simulink model "met_Lap_1_31"  (R2020b)
settings: Solver=VariableStepAuto  StartTime=0.0  StopTime=10.0  RelTol=1e-3
undefined symbols (not defined in the file): b, c, d, x0
libraries: simulink x1
settings Model: Creator=Hyperbook  LastModifiedBy=Hyperbook

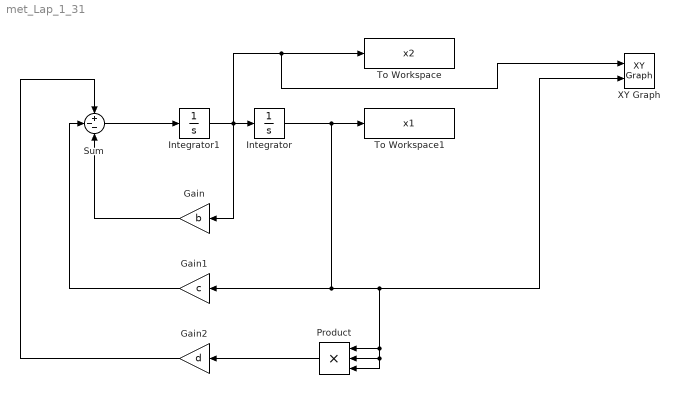
== system met_Lap_1_31 ==
  Gain : Gain  Gain=b
  Gain1 : Gain  Gain=c
  Gain2 : Gain  Gain=d
  Integrator : Integrator  InitialCondition=x0(2)  LimitOutput=on  UpperSaturationLimit=2  LowerSaturationLimit=-2
  Integrator1 : Integrator  InitialCondition=x0(1)  LimitOutput=on  UpperSaturationLimit=2  LowerSaturationLimit=-2
  Product : Product  Inputs=3
  Sum : Sum  Inputs=+--
  To Workspace : ToWorkspace  VariableName=x2  SampleTime=-1
  To Workspace1 : ToWorkspace  VariableName=x1  SampleTime=-1
  XY Graph : simulink/Sinks/XY Graph  xmin=-1  xmax=1  ymin=-1  ymax=1  st=-1
  wires:
  Integrator/1 -> XY Graph/2, Product/1, Product/3, Product/2, Gain1/1, To Workspace1/1
  Sum/1 -> Integrator1/1
  Gain/1 -> Sum/3
  Gain1/1 -> Sum/2
  Gain2/1 -> Sum/1
  Product/1 -> Gain2/1
  Integrator1/1 -> XY Graph/1, To Workspace/1, Gain/1, Integrator/1
